simulink subsystem "FuelCellSSC"  (R2024b)
settings: Solver=VariableStepAuto  StartTime=0.0  StopTime=10.0  RelTol=1e-3
undefined symbols (not defined in the file): EnvAirTemp, f_fc_auxpower, f_fc_currcmd_bpt, f_fc_h2flow, f_fc_heatflow, f_fc_tmpcmd_bpt, f_fc_voltage, HVDCNeg, HVDCPos, PlntBattNumCellSer, PlntBattOpenCirctVolt
libraries: fl_lib x15, nesl_utility x3, nesl_utility_internal x2, ee_lib x1, simulink x1, slpidlib x1
settings Model: ModifiedByFormat=The MathWorks, Inc.  Creator=The MathWorks, Inc.  LastModifiedBy=The MathWorks, Inc.
settings RTWCC: GPUComputeCapability=3.5

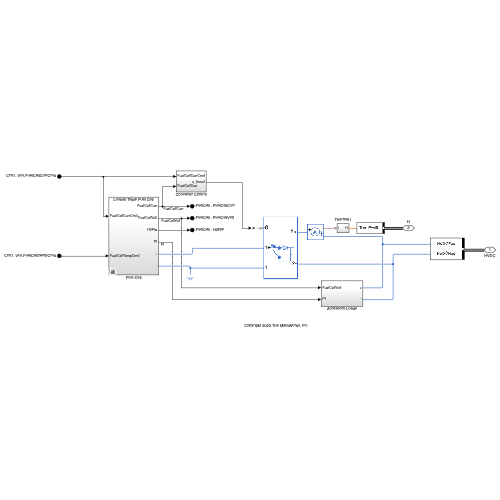
[thumbnail: Simulink's stored preview of the top-level diagram]
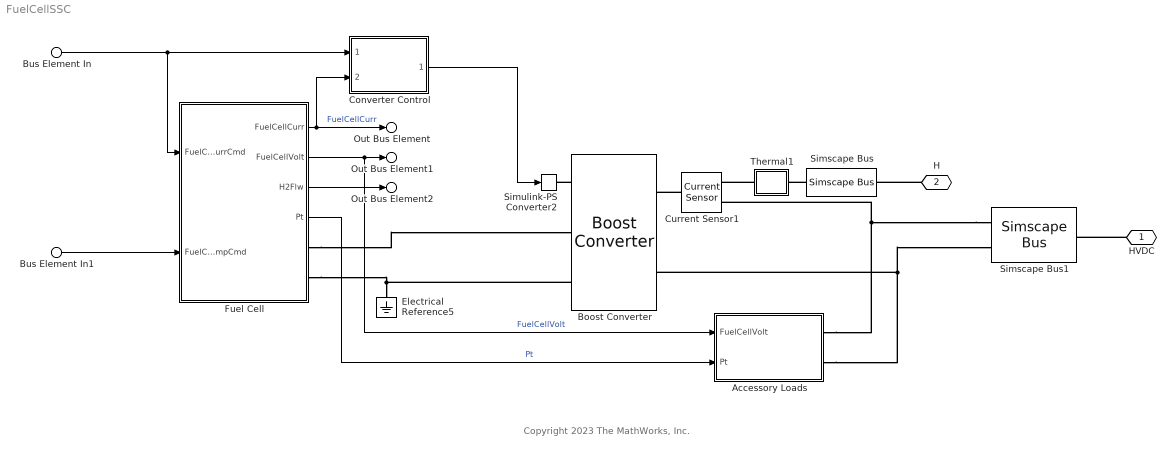
== system FuelCellSSC ==
  note: Copyright 2023 The MathWorks, Inc.
  Bus Element In : Inport  PortName=Cntrl  Element=Vcu.FuelCellCurrCmd
  Bus Element In1 : Inport  PortName=Cntrl  Element=Vcu.FuelCellTempCmd
  Accessory Loads : Subsystem
  Boost Converter : ee_lib/Semiconductors & Converters/Converters/Boost Converter  port_option=ee.enum.controlport.ps  device_type=ee.enum.converters.switchingdevice.averaged  Vf=0.8 V  Ron=FCDCDC.avgSwitchResistance Ohm  Rds=0.001 Ohm  Goff=1e-5 1/Ohm  Vgt=1 V  Vgt_off=-1 V  Ih=1 A  Vth=6 V  K=0  diode_param=ee.enum.converters.diode.nodynamics  diode_Vf=FCDCDC.diodeFwdVolt V  diode_Ron=FCDCDC.diodeOnResistance Ohm  diode_Goff=FCDCDC.diodeOffConductance 1/Ohm  diode_C=50 nF  diode_iRM=-235 A  diode_iF=300 A  diode_idot=-50 A/us  diode_trr_param=ee.enum.converters.diodetrr.trr_factor  diode_trr_factor=3  diode_trr=15 us  diode_Qrr=1500 s*uA  Lf=FCDCDC.inductance H  Rl=FCDCDC.inductorSeriesResistance Ohm  Cf=FCDCDC.capacitance F  Rf=FCDCDC.CapEffSeriesResistance Ohm  snubber_type=ee.enum.converters.snubber.exclude  Cs=1e-7 F  Rs=0.1 Ohm  iL_specify=on  iL_priority=High  iL=0 A  iL_nominal_specify=off  iL_nominal_value=1  iL_nominal_unit=A  vc_specify=on  vc_priority=High  vc=FCDCDC.Vout V  vc_nominal_specify=off  vc_nominal_value=1  vc_nominal_unit=V
      settings: InternalSimscapePortConfiguration="{\"Bottom\":[],\"Left\":[{\"id\":\"G\",\"label\":\"G\",\"type\":\"input\"},{\"id\":\"p1\",\"label\":\"1+\",\"type\":\"foundation.electrical.electrical\"},{\"id\":\"n1\",\"label\":\"1-\",\"type\":\"foundation.electrical.electrical\"}],\"Right\":[{\"id\":\"p2\",\"label\":\"2+\",\"type\":\"foundation.electrical.electrical\"},{\"id\":\"n2\",\"label\":\"2-\",\"type\":\"foundation.electrical.electrical\"}],\"Top\":[]}"
  Converter Control : Subsystem
  Current Sensor1 : fl_lib/Electrical/Electrical Sensors/Current Sensor
  Electrical Reference5 : fl_lib/Electrical/Electrical Elements/Electrical Reference
  Fuel Cell : Subsystem  Variant=on  VariantControlMode=label  VariantControl=Choice  LabelModeActiveChoice=Lookup Table Fuel Cell
  Simscape Bus : SimscapeBus  HierarchyStrings=ThrmPwrE1
  Simscape Bus1 : SimscapeBus  HierarchyStrings=HVDCPos;HVDCNeg
  Simulink-PS Converter2 : nesl_utility_internal/Simulink-PS Converter  PhysicalDomain=network_engine_domain  SubClassName=ps_input  LeftPortType=input  RightPortType=output  PseudoPeriodic=off  Frequencies=[]  NoiseDistribution=none  NoiseParameters=[]  Unit=1  AffineConversion=off  FilteringAndDerivatives=provide  SimscapeFilterOrder=1  InputFilterTimeConstant=0.001  UdotUserProvided=0
  Thermal1 : Subsystem
  HVDC : PMIOPort  Side=Right
  H : PMIOPort  Port=2  Side=Right
  Out Bus Element1 : Outport  PortName=FuelCell  Element=FuelCellVolt
  Out Bus Element : Outport  PortName=FuelCell  Element=FuelCellCurr
  Out Bus Element2 : Outport  PortName=FuelCell  Element=H2Flw
  wires:
  Fuel Cell/4(Pt) -> Accessory Loads/2(Pt)  "Pt"
  Converter Control/1(u_boost) -> Simulink-PS Converter2/1
  Fuel Cell/1(FuelCellCurr) -> Converter Control/2(FuelCellCurr), Out Bus Element/1  "FuelCellCurr"
  Fuel Cell/2(FuelCellVolt) -> Accessory Loads/1(FuelCellVolt), Out Bus Element1/1  "FuelCellVolt"
  Fuel Cell/3(H2Flw) -> Out Bus Element2/1
  Bus Element In/1 -> Converter Control/1(FuelCellCurrCmd), Fuel Cell/1(FuelCellCurrCmd)
  Bus Element In1/1 -> Fuel Cell/2(FuelCellTempCmd)
  connections:
  Boost Converter/RConn2 -- Accessory Loads/RConn2 -- Simscape Bus1/LConn2
  Simscape Bus1/LConn1 -- Accessory Loads/RConn1 -- Current Sensor1/RConn2
  Fuel Cell/RConn2 -- Boost Converter/LConn3 -- Electrical Reference5/LConn1
  Simscape Bus/LConn1 -- Thermal1/RConn1
  Boost Converter/LConn1 -- Simulink-PS Converter2/RConn1
  Current Sensor1/LConn1 -- Boost Converter/RConn1
  Thermal1/LConn1 -- Current Sensor1/RConn1
  H/RConn1 -- Simscape Bus/RConn1
  Fuel Cell/RConn1 -- Boost Converter/LConn2
  HVDC/RConn1 -- Simscape Bus1/RConn1

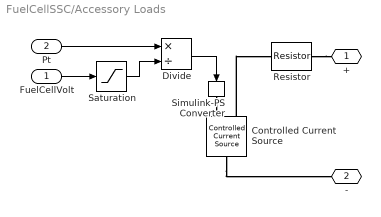
== system FuelCellSSC/Accessory Loads ==
  FuelCellVolt : Inport
  Pt : Inport  Port=2
  Controlled Current Source : fl_lib/Electrical/Electrical Sources/Controlled Current Source
  Divide : Product  Inputs=*/
  Resistor : fl_lib/Electrical/Electrical Elements/Resistor  R=1e-6 Ohm  i_specify=off  i_priority=None  i=0 A  i_nominal_specify=off  i_nominal_value=1  i_nominal_unit=A  v_specify=off  v_priority=None  v=0 V  v_nominal_specify=off  v_nominal_value=1  v_nominal_unit=V
  Saturation : Saturate  UpperLimit=inf  LowerLimit=min(PlntBattOpenCirctVolt, [], 'all')*PlntBattNumCellSer  ZeroCross=off
  Simulink-PS Converter : nesl_utility_internal/Simulink-PS Converter  PhysicalDomain=network_engine_domain  SubClassName=ps_input  LeftPortType=input  RightPortType=output  PseudoPeriodic=off  Frequencies=[]  NoiseDistribution=none  NoiseParameters=[]  Unit=A  AffineConversion=off  FilteringAndDerivatives=provide  SimscapeFilterOrder=1  InputFilterTimeConstant=0.001  UdotUserProvided=0
  + : PMIOPort  Side=Right
  - : PMIOPort  Port=2  Side=Right
  wires:
  Pt/1 -> Divide/1
  Divide/1 -> Simulink-PS Converter/1
  Saturation/1 -> Divide/2
  FuelCellVolt/1 -> Saturation/1
  connections:
  Simulink-PS Converter/RConn1 -- Controlled Current Source/RConn1
  Controlled Current Source/LConn1 -- -/RConn1
  Controlled Current Source/RConn2 -- Resistor/RConn1
  Resistor/LConn1 -- +/RConn1

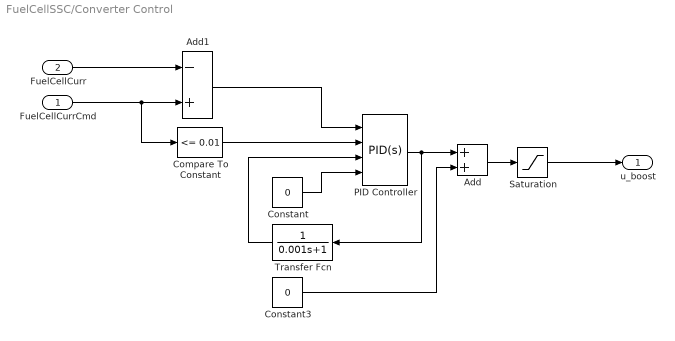
== system FuelCellSSC/Converter Control ==
  FuelCellCurrCmd : Inport
  FuelCellCurr : Inport  Port=2
  Add : Sum
  Add1 : Sum  Inputs=-+
  Compare To Constant : simulink/Logic and Bit Operations/Compare To Constant  relop=<=  const=0.01  OutDataTypeStr=boolean  ZeroCross=off
  Constant : Constant  Value=0  SampleTime=-1
  Constant3 : Constant  Value=0  SampleTime=-1
  PID Controller : slpidlib/PID Controller  Controller=PID  Form=Parallel  TimeDomain=Continuous-time  UseExternalTs=off  SampleTime=-1  IntegratorMethod=Forward Euler  FilterMethod=Forward Euler  ControllerParametersSource=internal  P=0.006  I=0.01  UseKiTs=off  D=0  UseExternalDerivativeSource=off  N=100  UseFilter=on  TunerSelectOption=Transfer Function Based (PID Tuner App)  ZeroCross=off  InitialConditionSource=external  InitialConditionForIntegrator=0  InitialConditionForFilter=0  DifferentiatorICPrevScaledInput=0  ExternalReset=falling  TrackingMode=off  Kt=1  LimitOutput=on  SatLimitsSource=internal  UpperSaturationLimit=1  LowerSaturationLimit=-1  LinearizeAsGain=on  AntiWindupMode=none  Kb=1  LimitIntegrator=off  UpperIntegratorSaturationLimit=inf  LowerIntegratorSaturationLimit=-inf  POutMin=[]  POutMax=[]  IOutMin=[]  IOutMax=[]  DOutMin=[]  DOutMax=[]  NOutMin=[]  NOutMax=[]  SumOutMin=[]  SumOutMax=[]  SaturationOutMin=[]  SaturationOutMax=[]  PParamMin=[]  PParamMax=[]  IParamMin=[]  IParamMax=[]  DParamMin=[]  DParamMax=[]  NParamMin=[]  NParamMax=[]  KbParamMin=[]  KbParamMax=[]  KtParamMin=[]  KtParamMax=[]  KbOutMin=[]  KbOutMax=[]  KtOutMin=[]  KtOutMax=[]  IntegratorOutMin=[]  IntegratorOutMax=[]  FilterOutMin=[]  FilterOutMax=[]  SumI1OutMin=[]  SumI1OutMax=[]  SumI2OutMin=[]  SumI2OutMax=[]  SumI3OutMin=[]  SumI3OutMax=[]  SumI4OutMin=[]  SumI4OutMax=[]  SumDOutMin=[]  SumDOutMax=[]  DifferentiatorOutMin=[]  DifferentiatorOutMax=[]  FilterDiffOutCoefMin=[]  FilterDiffOutCoefMax=[]  ReciprocalOutMin=[]  ReciprocalOutMax=[]  SumDenOutMin=[]  SumDenOutMax=[]  SumNumOutMin=[]  SumNumOutMax=[]  DivideOutMin=[]  DivideOutMax=[]  UdiffTsProdOutMin=[]  UdiffTsProdOutMax=[]  NTsProdOutMin=[]  NTsProdOutMax=[]  UintegralTsProdOutMin=[]  UintegralTsProdOutMax=[]  UngainTsProdOutMin=[]  UngainTsProdOutMax=[]  ClampingZeroOutDataTypeStr=Inherit: Inherit via back propagation  ClampingZeroOutMin=[]  ClampingZeroOutMax=[]  FilterDenConstantOutDataTypeStr=Inherit: Inherit via back propagation  FilterDenConstantOutMin=[]  FilterDenConstantOutMax=[]  PCopyOutDataTypeStr=Inherit: Inherit via back propagation  PCopyOutMin=[]  PCopyOutMax=[]  NCopyOutDataTypeStr=Inherit: Inherit via back propagation  NCopyOutMin=[]  NCopyOutMax=[]  IntegratorContinuousStateAttributes=''  IntegratorStateMustResolveToSignalObject=off  IntegratorRTWStateStorageClass=Auto  FilterContinuousStateAttributes=''  FilterStateMustResolveToSignalObject=off  FilterRTWStateStorageClass=Auto  ParallelPVariant=InternalParameters  IdealPVariant=Disabled  IVariant=InternalParameters  DVariant=InternalParameters  IntegratorVariant=Continuous  SatVariant=Enabled  AWVariant=Passthrough  PCopyVariant=Disabled  TRVariant=Disabled  FdbkBlocksVariant=Forward  IdealPFdbkVariant=Disabled  SatFdbkVariant=Disabled  DerivativeFilterVariant=ContFilter  NVariant=InternalParameters  NCopyVariant=Disabled  FilterICVariant=ExternalICs  IntegratorICVariant=ExternalICs  ExternalResetVariant=ExternalReset  TRSumVariant=Passthrough  SumFdbkVariant=Disabled  SumVariant=Sum_PID  TsampFilterVariant=InternalTs  TsampNgainVariant=Passthrough  TsampIntegralVariant=Disabled_SignalSpec  ExternalSaturationOutDataTypeStr=Inherit: Same as second input  DerivativeSourceVariant=ErrorSignal  PreIntVariant=InternalPreInt
  Saturation : Saturate  UpperLimit=1  LowerLimit=0
  Transfer Fcn : TransferFcn  Denominator=[0.001 1]
  u_boost : Outport
  wires:
  Saturation/1 -> u_boost/1
  Compare To Constant/1 -> PID Controller/2
  Constant/1 -> PID Controller/4
  Transfer Fcn/1 -> PID Controller/3
  Add1/1 -> PID Controller/1
  FuelCellCurrCmd/1 -> Add1/2, Compare To Constant/1
  Add/1 -> Saturation/1
  FuelCellCurr/1 -> Add1/1
  PID Controller/1 -> Transfer Fcn/1, Add/1
  Constant3/1 -> Add/2

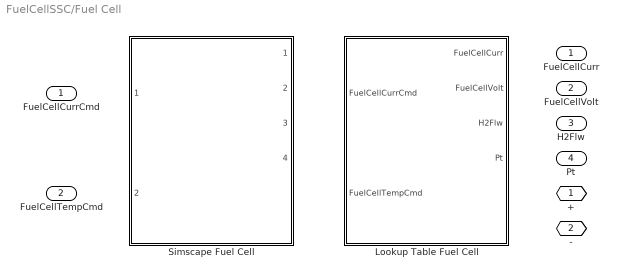
== system FuelCellSSC/Fuel Cell ==
  FuelCellCurrCmd : Inport
  FuelCellTempCmd : Inport  Port=2
  Lookup Table Fuel Cell : Subsystem  VariantControl=Lookup Table Fuel Cell
  Simscape Fuel Cell : Subsystem  VariantControl=Simscape Fuel Cell  ReferencedSubsystem=FuelCellCore
  + : PMIOPort  Side=Right
  - : PMIOPort  Port=2  Side=Right
  FuelCellCurr : Outport
  FuelCellVolt : Outport  Port=2
  H2Flw : Outport  Port=3
  Pt : Outport  Port=4

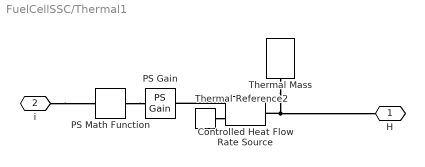
== system FuelCellSSC/Thermal1 ==
  Controlled Heat Flow Rate Source : fl_lib/Thermal/Thermal Sources/Controlled Heat Flow Rate Source
  PS Gain : fl_lib/Physical Signals/Functions/PS Gain  gain=0.001 Ohm
  PS Math Function : fl_lib/Physical Signals/Functions/PS Math Function  fcn_choice=foundation.enum.math_function.square  v=1
  Thermal Mass : fl_lib/Thermal/Thermal Elements/Thermal Mass  mass_type=foundation.enum.constant_variable.constant  mass=500 kg  sp_heat=447 J/kg/K  mass_min=1e-6 kg  num_ports=foundation.enum.numPorts2.one  m_specify=off  m_priority=High  m=1 kg  m_nominal_specify=off  m_nominal_value=1  m_nominal_unit=kg  T_specify=on  T_priority=High  T=EnvAirTemp K  T_nominal_specify=off  T_nominal_value=1  T_nominal_unit=K  Q_specify=off  Q_priority=None  Q=0 W  Q_nominal_specify=off  Q_nominal_value=1  Q_nominal_unit=W
  Thermal Reference2 : fl_lib/Thermal/Thermal Elements/Thermal Reference
  H : PMIOPort  Side=Right
  i : PMIOPort  Port=2  Side=Left
  connections:
  Controlled Heat Flow Rate Source/RConn1 -- PS Gain/RConn1
  PS Math Function/RConn1 -- PS Gain/LConn1
  Thermal Reference2/LConn1 -- Controlled Heat Flow Rate Source/RConn2
  i/RConn1 -- PS Math Function/LConn1
  Thermal Mass/LConn1 -- Controlled Heat Flow Rate Source/LConn1 -- H/RConn1

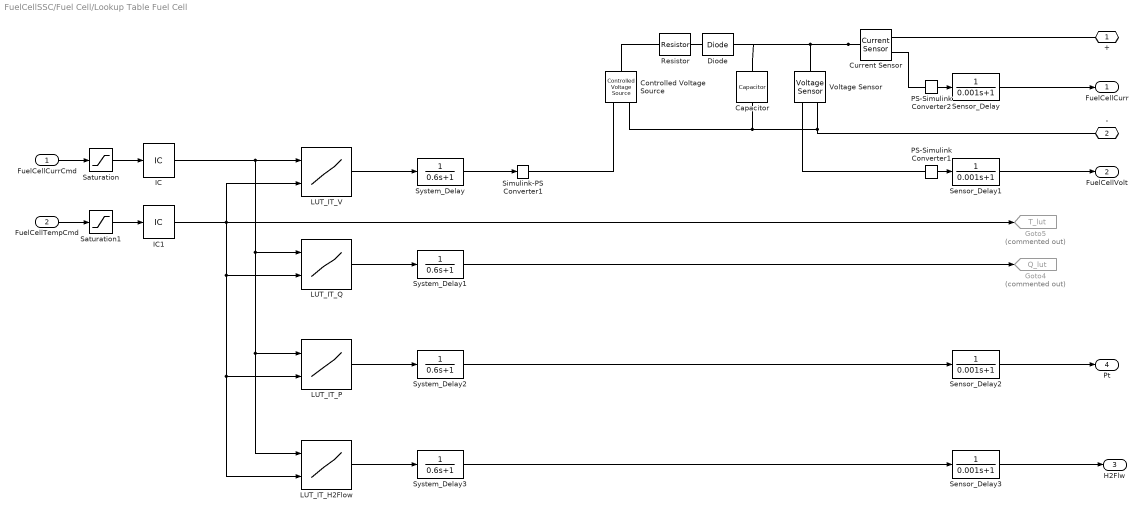
== system FuelCellSSC/Fuel Cell/Lookup Table Fuel Cell ==
  FuelCellCurrCmd : Inport
  FuelCellTempCmd : Inport  Port=2
  Capacitor : fl_lib/Electrical/Electrical Elements/Capacitor  c=1e-6 F  r=1e-6 Ohm  g=0 1/Ohm  i_specify=off  i_priority=None  i=0 A  i_nominal_specify=off  i_nominal_value=1  i_nominal_unit=A  v_specify=off  v_priority=None  v=0 V  v_nominal_specify=off  v_nominal_value=1  v_nominal_unit=V  vc_specify=on  vc_priority=High  vc=f_fc_voltage(1) V  vc_nominal_specify=off  vc_nominal_value=1  vc_nominal_unit=V
  Controlled Voltage Source : fl_lib/Electrical/Electrical Sources/Controlled Voltage Source
  Current Sensor : fl_lib/Electrical/Electrical Sensors/Current Sensor
  Diode : fl_lib/Electrical/Electrical Elements/Diode  Vf=0.6 V  Ron=0.3 Ohm  Goff=1e-8 1/Ohm  i_specify=off  i_priority=None  i=0 A  i_nominal_specify=off  i_nominal_value=1  i_nominal_unit=A  v_specify=off  v_priority=None  v=0 V  v_nominal_specify=off  v_nominal_value=1  v_nominal_unit=V
  Goto4 : Goto  Commented=on  GotoTag=Q_lut  TagVisibility=global
  Goto5 : Goto  Commented=on  GotoTag=T_lut  TagVisibility=global
  IC : InitialCondition  Value=f_fc_currcmd_bpt(1)
  IC1 : InitialCondition  Value=f_fc_tmpcmd_bpt(1)
  LUT_IT_H2Flow : Lookup_n-D  BreakpointsForDimension1=f_fc_currcmd_bpt  BreakpointsForDimension2=f_fc_tmpcmd_bpt  Table=f_fc_h2flow  InternalRulePriority=Speed  RndMeth=Simplest
      settings: InputPortMap=u0,u1
  LUT_IT_P : Lookup_n-D  BreakpointsForDimension1=f_fc_currcmd_bpt  BreakpointsForDimension2=f_fc_tmpcmd_bpt  Table=f_fc_auxpower  InternalRulePriority=Speed  RndMeth=Simplest
      settings: InputPortMap=u0,u1
  LUT_IT_Q : Lookup_n-D  BreakpointsForDimension1=f_fc_currcmd_bpt  BreakpointsForDimension2=f_fc_tmpcmd_bpt  Table=f_fc_heatflow  InternalRulePriority=Speed  RndMeth=Simplest
      settings: InputPortMap=u0,u1
  LUT_IT_V : Lookup_n-D  BreakpointsForDimension1=f_fc_currcmd_bpt  BreakpointsForDimension2=f_fc_tmpcmd_bpt  Table=f_fc_voltage  InternalRulePriority=Speed  RndMeth=Simplest
      settings: InputPortMap=u0,u1
  PS-Simulink Converter1 : nesl_utility/PS-Simulink Converter  PhysicalDomain=network_engine_domain  SubClassName=ps_output  LeftPortType=input  RightPortType=output  PseudoPeriodic=off  Frequencies=[]  VectorFormat=1-D array  Unit=inherit  AffineConversion=off
  PS-Simulink Converter2 : nesl_utility/PS-Simulink Converter  PhysicalDomain=network_engine_domain  SubClassName=ps_output  LeftPortType=input  RightPortType=output  PseudoPeriodic=off  Frequencies=[]  VectorFormat=1-D array  Unit=1  AffineConversion=off
  Resistor : fl_lib/Electrical/Electrical Elements/Resistor  R=1e-3 Ohm  i_specify=off  i_priority=None  i=0 A  i_nominal_specify=off  i_nominal_value=1  i_nominal_unit=A  v_specify=off  v_priority=None  v=0 V  v_nominal_specify=off  v_nominal_value=1  v_nominal_unit=V
  Saturation : Saturate  UpperLimit=max(f_fc_currcmd_bpt)  LowerLimit=0
  Saturation1 : Saturate  UpperLimit=max(f_fc_tmpcmd_bpt)  LowerLimit=0
  Sensor_Delay{,1..3} (4 alike) : TransferFcn  Denominator=[0.001 1]
  Simulink-PS Converter1 : nesl_utility/Simulink-PS Converter  PhysicalDomain=network_engine_domain  SubClassName=ps_input  LeftPortType=input  RightPortType=output  PseudoPeriodic=off  Frequencies=[]  NoiseDistribution=none  NoiseParameters=[]  Unit=V  AffineConversion=off  FilteringAndDerivatives=provide  SimscapeFilterOrder=1  InputFilterTimeConstant=0.001  UdotUserProvided=0
  System_Delay{,1..3} (4 alike) : TransferFcn  Denominator=[0.6 1]
  Voltage Sensor : fl_lib/Electrical/Electrical Sensors/Voltage Sensor
  + : PMIOPort  Side=Right
  - : PMIOPort  Port=2  Side=Right
  FuelCellCurr : Outport
  FuelCellVolt : Outport  Port=2
  H2Flw : Outport  Port=3
  Pt : Outport  Port=4
  wires:
  System_Delay2/1 -> Sensor_Delay2/1
  System_Delay1/1 -> Goto4/1
  LUT_IT_Q/1 -> System_Delay1/1
  LUT_IT_V/1 -> System_Delay/1
  IC1/1 -> LUT_IT_V/2, Goto5/1, LUT_IT_H2Flow/2, LUT_IT_P/2, LUT_IT_Q/2
  Saturation/1 -> IC/1
  PS-Simulink Converter2/1 -> Sensor_Delay/1
  PS-Simulink Converter1/1 -> Sensor_Delay1/1
  LUT_IT_P/1 -> System_Delay2/1
  Saturation1/1 -> IC1/1
  LUT_IT_H2Flow/1 -> System_Delay3/1
  IC/1 -> LUT_IT_H2Flow/1, LUT_IT_P/1, LUT_IT_Q/1, LUT_IT_V/1
  System_Delay3/1 -> Sensor_Delay3/1
  System_Delay/1 -> Simulink-PS Converter1/1
  FuelCellCurrCmd/1 -> Saturation/1
  FuelCellTempCmd/1 -> Saturation1/1
  Sensor_Delay2/1 -> Pt/1
  Sensor_Delay3/1 -> H2Flw/1
  Sensor_Delay1/1 -> FuelCellVolt/1
  Sensor_Delay/1 -> FuelCellCurr/1
  connections:
  Current Sensor/LConn1 -- Voltage Sensor/LConn1 -- Diode/RConn1 -- Capacitor/LConn1
  Controlled Voltage Source/RConn2 -- Capacitor/RConn1 -- Voltage Sensor/RConn2 -- -/RConn1
  +/RConn1 -- Current Sensor/RConn2
  PS-Simulink Converter1/LConn1 -- Voltage Sensor/RConn1
  Controlled Voltage Source/LConn1 -- Resistor/LConn1
  PS-Simulink Converter2/LConn1 -- Current Sensor/RConn1
  Resistor/RConn1 -- Diode/LConn1
  Simulink-PS Converter1/RConn1 -- Controlled Voltage Source/RConn1
